simulink model "smc_2"  (R2017a)
settings: Solver=FixedStepAuto  StartTime=0.0  StopTime=100  FixedStep=0.001  RelTol=1e-3
undefined symbols (not defined in the file): A, c, k, psi, sin_input, w, x01, x02
settings Model: Creator=Matteo  LastModifiedBy=Matteo

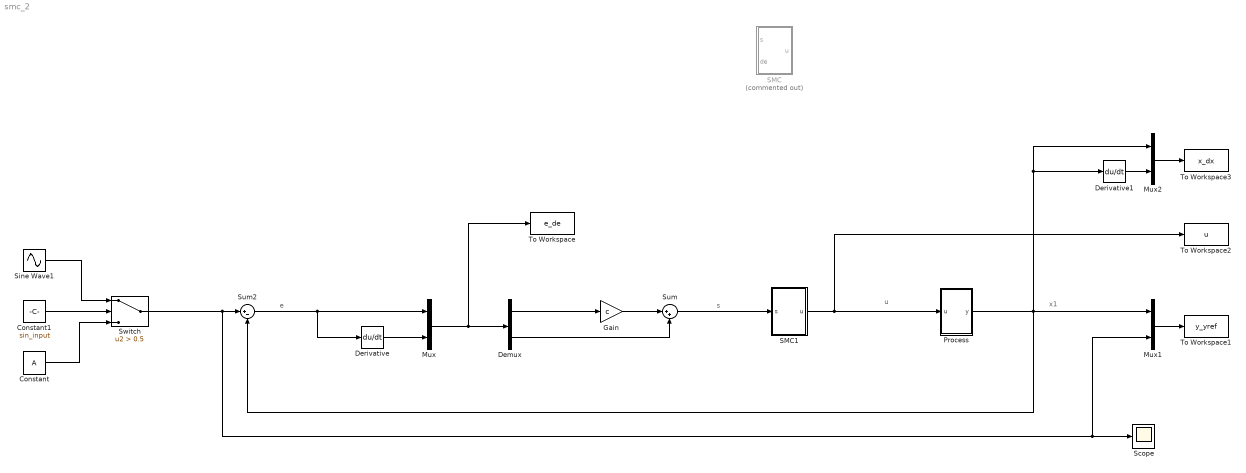
== system smc_2 ==
  note: e
  note: s
  note: x1
  note: u
  Constant : Constant  Value=A
  Constant1 : Constant  Value=sin_input
  Demux : Demux  Outputs=2
  Derivative : Derivative
  Derivative1 : Derivative
  Gain : Gain  Gain=c
  Mux : Mux  Inputs=2
  Mux1 : Mux  Inputs=2
  Mux2 : Mux  Inputs=2
  Process : Subsystem
  SMC : Subsystem  Commented=on
  SMC1 : Subsystem
  Scope : Scope
  Sine Wave1 : Sin  Amplitude=A  Frequency=w  SampleTime=0
  Sum : Sum  Inputs=|++
  Sum2 : Sum  Inputs=|+-
  Switch : Switch  Criteria=u2 > Threshold  Threshold=0.5
  To Workspace : ToWorkspace  VariableName=e_de  SampleTime=-1
  To Workspace1 : ToWorkspace  VariableName=y_yref  SaveFormat=Structure With Time  SampleTime=-1
  To Workspace2 : ToWorkspace  VariableName=u  SaveFormat=Structure With Time  SampleTime=-1
  To Workspace3 : ToWorkspace  VariableName=x_dx  SampleTime=-1
  wires:
  Derivative/1 -> Mux/2
  Mux/1 -> To Workspace/1, Demux/1
  Sum2/1 -> Derivative/1, Mux/1
  Demux/1 -> Gain/1
  Gain/1 -> Sum/1
  Demux/2 -> Sum/2
  Mux1/1 -> To Workspace1/1
  Switch/1 -> Mux1/2, Scope/1, Sum2/1
  Derivative1/1 -> Mux2/2
  Mux2/1 -> To Workspace3/1
  Sine Wave1/1 -> Switch/1
  Constant/1 -> Switch/3
  SMC1/1(u) -> To Workspace2/1, Process/1(u)
  Sum/1 -> SMC1/1(s)
  Constant1/1 -> Switch/2
  Process/1(y) -> Derivative1/1, Mux2/1, Sum2/2, Mux1/1

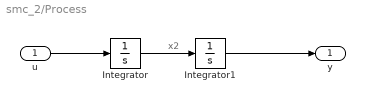
== system smc_2/Process ==
  note: x2
  u : Inport
  Integrator : Integrator  InitialCondition=x02
  Integrator1 : Integrator  InitialCondition=x01
  y : Outport
  wires:
  u/1 -> Integrator/1
  Integrator1/1 -> y/1
  Integrator/1 -> Integrator1/1

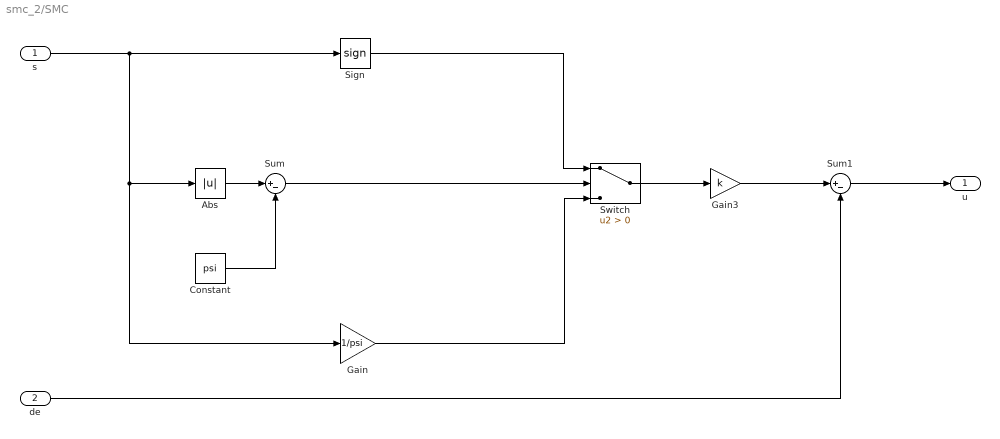
== system smc_2/SMC ==
  s : Inport
  de : Inport  Port=2
  Abs : Abs  ZeroCross=off
  Constant : Constant  Value=psi
  Gain : Gain  Gain=1/psi
  Gain3 : Gain  Gain=k
  Sign : Signum  ZeroCross=off
  Sum : Sum  Inputs=|+-
  Sum1 : Sum  Inputs=|+-
  Switch : Switch  Criteria=u2 > Threshold  ZeroCross=off
  u : Outport
  wires:
  Sum/1 -> Switch/2
  Abs/1 -> Sum/1
  Constant/1 -> Sum/2
  Sign/1 -> Switch/1
  Switch/1 -> Gain3/1
  Gain3/1 -> Sum1/1
  s/1 -> Sign/1, Abs/1, Gain/1
  Gain/1 -> Switch/3
  de/1 -> Sum1/2
  Sum1/1 -> u/1

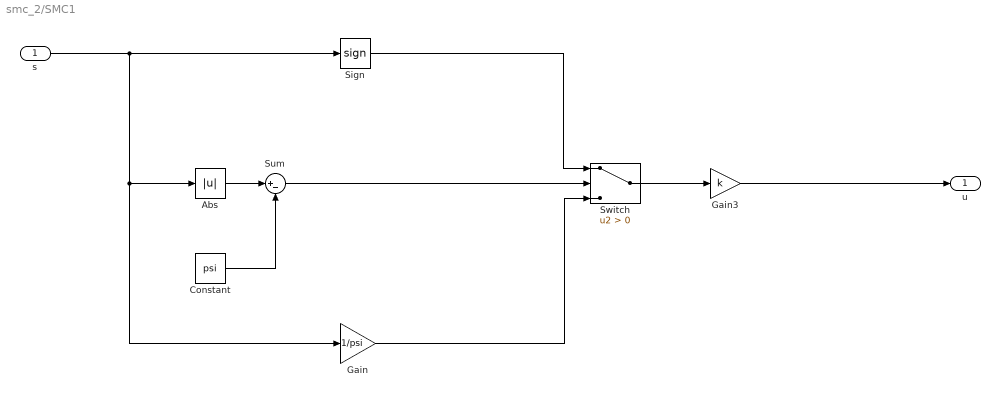
== system smc_2/SMC1 ==
  s : Inport
  Abs : Abs  ZeroCross=off
  Constant : Constant  Value=psi
  Gain : Gain  Gain=1/psi
  Gain3 : Gain  Gain=k
  Sign : Signum  ZeroCross=off
  Sum : Sum  Inputs=|+-
  Switch : Switch  Criteria=u2 > Threshold  ZeroCross=off
  u : Outport
  wires:
  Sum/1 -> Switch/2
  Abs/1 -> Sum/1
  Constant/1 -> Sum/2
  Sign/1 -> Switch/1
  Switch/1 -> Gain3/1
  s/1 -> Sign/1, Abs/1, Gain/1
  Gain/1 -> Switch/3
  Gain3/1 -> u/1
